simulink model "power_microgrid_v5_battery"  (R2018b)
settings: Solver=ode23tb  StartTime=0.0  StopTime=24*60*60  FixedStep=1/(1000)  MaxStep=60  RelTol=1e-4
PreLoadFcn:
  | load('solar_load_data_24h.mat')
PostLoadFcn:
  | data = xlsread('Domestic_data_all_x3','Sheet1');
  | breakpoints1 = data(2:end,1)'
  | breakpoints2 = data(1,2:end)
  | table_data = data(2:end,2:end)
values from neighbouring files (symbols this model uses):
  SPD_1min = [0 0 0 0 0 0 0 0 0 0 0 0 ... (1441 elements, 1441x1)]    [default_PV_data.mat]
  SPT_1min = [0 60 120 180 240 300 360 420 480 540 600 660 ... (1441 elements, 1441x1)]    [default_PV_data.mat]
libraries: powerlib x155
(part 5 of 5)

== system power_microgrid_v5_battery/PV1 ==
  Clock : Clock
  Complex to Magnitude-Angle : ComplexToMagnitudeAngle  Output=Angle
  Controlled Current Source : powerlib/Electrical Sources/Controlled Current Source  Initialize=on  Source_Type=AC  Amplitude=0  Phase=0  Frequency=50  Measurements=None
      settings: SourceProductName=Simscape Electrical
  Gain10 : Gain  Gain=sqrt(2)
  Gain5 : Gain  Gain=1/230
  Ground2 : powerlib/Elements/Ground  LConnTagsString=a
      settings: SourceProductName=Simscape Electrical
  Magnitude-Angle to Complex1 : MagnitudeAngleToComplex
  Snubber1 : powerlib/Elements/Series RLC Branch  LConnTagsString=__new0  RConnTagsString=__new0  BranchType=R  Resistance=1e6  Inductance=1e-3  SetiL0=off  InitialCurrent=0  Capacitance=1e-6  Setx0=off  InitialVoltage=0  Measurements=None
      settings: SourceProductName=Simscape Electrical
  Solar Data 1-D Lookup Table : Lookup_n-D  NumberOfTableDimensions=1  BreakpointsForDimension1=SPT_1min  BeginIndexSearchUsingPreviousIndexResult=on  Table=SPD_1min  InternalRulePriority=Speed  RndMeth=Simplest  InputSameDT=on
  meas cur3 : powerlib/Measurements/Current Measurement  PhasorSimulation=on  OutputType=Complex  PSBequivalent=0
      settings: SourceProductName=Simscape Electrical
  Conn1 : PMIOPort  Side=Left
  Out1 : Outport
  wires:
  meas cur3/1 -> Out1/1
  Magnitude-Angle to Complex1/1 -> Controlled Current Source/1
  Clock/1 -> Solar Data 1-D Lookup Table/1
  Solar Data 1-D Lookup Table/1 -> Gain5/1
  Gain5/1 -> Gain10/1
  Gain10/1 -> Magnitude-Angle to Complex1/1
  Complex to Magnitude-Angle/1 -> Magnitude-Angle to Complex1/2
  [Vsec] -> Complex to Magnitude-Angle/1
  connections:
  Ground2/LConn1 -- Controlled Current Source/LConn1 -- Snubber1/RConn1
  Snubber1/LConn1 -- Controlled Current Source/RConn1 -- meas cur3/LConn1
  Conn1/RConn1 -- meas cur3/RConn1

== system power_microgrid_v5_battery/PV2 ==
  Clock : Clock
  Complex to Magnitude-Angle : ComplexToMagnitudeAngle  Output=Angle
  Controlled Current Source : powerlib/Electrical Sources/Controlled Current Source  Initialize=on  Source_Type=AC  Amplitude=0  Phase=0  Frequency=50  Measurements=None
      settings: SourceProductName=Simscape Electrical
  Gain10 : Gain  Gain=sqrt(2)
  Gain5 : Gain  Gain=1/230
  Ground2 : powerlib/Elements/Ground  LConnTagsString=a
      settings: SourceProductName=Simscape Electrical
  Magnitude-Angle to Complex1 : MagnitudeAngleToComplex
  Snubber1 : powerlib/Elements/Series RLC Branch  LConnTagsString=__new0  RConnTagsString=__new0  BranchType=R  Resistance=1e6  Inductance=1e-3  SetiL0=off  InitialCurrent=0  Capacitance=1e-6  Setx0=off  InitialVoltage=0  Measurements=None
      settings: SourceProductName=Simscape Electrical
  Solar Data 1-D Lookup Table : Lookup_n-D  NumberOfTableDimensions=1  BreakpointsForDimension1=SPT_1min  BeginIndexSearchUsingPreviousIndexResult=on  Table=SPD_1min  InternalRulePriority=Speed  RndMeth=Simplest  InputSameDT=on
  meas cur3 : powerlib/Measurements/Current Measurement  PhasorSimulation=on  OutputType=Complex  PSBequivalent=0
      settings: SourceProductName=Simscape Electrical
  Conn1 : PMIOPort  Side=Left
  Out1 : Outport
  wires:
  meas cur3/1 -> Out1/1
  Magnitude-Angle to Complex1/1 -> Controlled Current Source/1
  Clock/1 -> Solar Data 1-D Lookup Table/1
  Solar Data 1-D Lookup Table/1 -> Gain5/1
  Gain5/1 -> Gain10/1
  Gain10/1 -> Magnitude-Angle to Complex1/1
  Complex to Magnitude-Angle/1 -> Magnitude-Angle to Complex1/2
  [Vsec] -> Complex to Magnitude-Angle/1
  connections:
  Ground2/LConn1 -- Controlled Current Source/LConn1 -- Snubber1/RConn1
  Snubber1/LConn1 -- Controlled Current Source/RConn1 -- meas cur3/LConn1
  Conn1/RConn1 -- meas cur3/RConn1

== system power_microgrid_v5_battery/PV3 ==
  Clock : Clock
  Complex to Magnitude-Angle : ComplexToMagnitudeAngle  Output=Angle
  Controlled Current Source : powerlib/Electrical Sources/Controlled Current Source  Initialize=on  Source_Type=AC  Amplitude=0  Phase=0  Frequency=50  Measurements=None
      settings: SourceProductName=Simscape Electrical
  Gain10 : Gain  Gain=sqrt(2)
  Gain5 : Gain  Gain=1/230
  Ground2 : powerlib/Elements/Ground  LConnTagsString=a
      settings: SourceProductName=Simscape Electrical
  Magnitude-Angle to Complex1 : MagnitudeAngleToComplex
  Snubber1 : powerlib/Elements/Series RLC Branch  LConnTagsString=__new0  RConnTagsString=__new0  BranchType=R  Resistance=1e6  Inductance=1e-3  SetiL0=off  InitialCurrent=0  Capacitance=1e-6  Setx0=off  InitialVoltage=0  Measurements=None
      settings: SourceProductName=Simscape Electrical
  Solar Data 1-D Lookup Table : Lookup_n-D  NumberOfTableDimensions=1  BreakpointsForDimension1=SPT_1min  BeginIndexSearchUsingPreviousIndexResult=on  Table=SPD_1min  InternalRulePriority=Speed  RndMeth=Simplest  InputSameDT=on
  meas cur3 : powerlib/Measurements/Current Measurement  PhasorSimulation=on  OutputType=Complex  PSBequivalent=0
      settings: SourceProductName=Simscape Electrical
  Conn1 : PMIOPort  Side=Left
  Out1 : Outport
  wires:
  meas cur3/1 -> Out1/1
  Magnitude-Angle to Complex1/1 -> Controlled Current Source/1
  Clock/1 -> Solar Data 1-D Lookup Table/1
  Solar Data 1-D Lookup Table/1 -> Gain5/1
  Gain5/1 -> Gain10/1
  Gain10/1 -> Magnitude-Angle to Complex1/1
  Complex to Magnitude-Angle/1 -> Magnitude-Angle to Complex1/2
  [Vsec] -> Complex to Magnitude-Angle/1
  connections:
  Ground2/LConn1 -- Controlled Current Source/LConn1 -- Snubber1/RConn1
  Snubber1/LConn1 -- Controlled Current Source/RConn1 -- meas cur3/LConn1
  Conn1/RConn1 -- meas cur3/RConn1

== system power_microgrid_v5_battery/PV4 ==
  Clock : Clock
  Complex to Magnitude-Angle : ComplexToMagnitudeAngle  Output=Angle
  Controlled Current Source : powerlib/Electrical Sources/Controlled Current Source  Initialize=on  Source_Type=AC  Amplitude=0  Phase=0  Frequency=50  Measurements=None
      settings: SourceProductName=Simscape Electrical
  Gain10 : Gain  Gain=sqrt(2)
  Gain5 : Gain  Gain=2/230
  Ground2 : powerlib/Elements/Ground  LConnTagsString=a
      settings: SourceProductName=Simscape Electrical
  Magnitude-Angle to Complex1 : MagnitudeAngleToComplex
  Snubber1 : powerlib/Elements/Series RLC Branch  LConnTagsString=__new0  RConnTagsString=__new0  BranchType=R  Resistance=1e6  Inductance=1e-3  SetiL0=off  InitialCurrent=0  Capacitance=1e-6  Setx0=off  InitialVoltage=0  Measurements=None
      settings: SourceProductName=Simscape Electrical
  Solar Data 1-D Lookup Table : Lookup_n-D  NumberOfTableDimensions=1  BreakpointsForDimension1=SPT_1min  BeginIndexSearchUsingPreviousIndexResult=on  Table=SPD_1min  InternalRulePriority=Speed  RndMeth=Simplest  InputSameDT=on
  meas cur3 : powerlib/Measurements/Current Measurement  PhasorSimulation=on  OutputType=Complex  PSBequivalent=0
      settings: SourceProductName=Simscape Electrical
  Conn1 : PMIOPort  Side=Left
  Out1 : Outport
  wires:
  meas cur3/1 -> Out1/1
  Magnitude-Angle to Complex1/1 -> Controlled Current Source/1
  Clock/1 -> Solar Data 1-D Lookup Table/1
  Solar Data 1-D Lookup Table/1 -> Gain5/1
  Gain5/1 -> Gain10/1
  Gain10/1 -> Magnitude-Angle to Complex1/1
  Complex to Magnitude-Angle/1 -> Magnitude-Angle to Complex1/2
  [Vsec] -> Complex to Magnitude-Angle/1
  connections:
  Ground2/LConn1 -- Controlled Current Source/LConn1 -- Snubber1/RConn1
  Snubber1/LConn1 -- Controlled Current Source/RConn1 -- meas cur3/LConn1
  Conn1/RConn1 -- meas cur3/RConn1

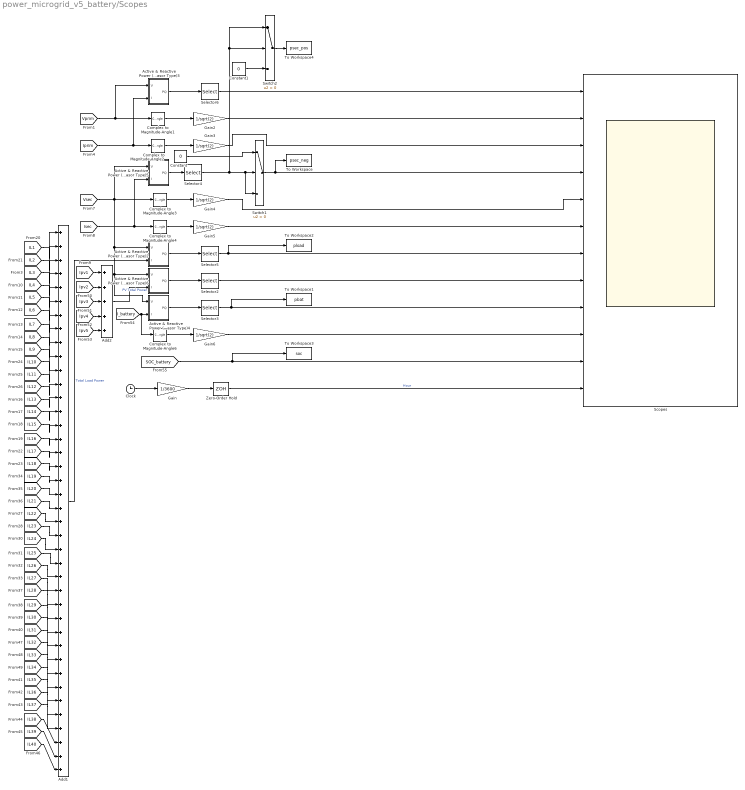
== system power_microgrid_v5_battery/Scopes ==
  Active & Reactive Power (Phasor Type)2 : Subsystem  DialogController=POWERSYS.PowerSysDialog  mask(Active & Reactive Power (Phasor Type)){}
      mask help: Active & Reactive Power (Phasor Type)
      mask init:
      | power_initmask();
      mask Help: This block is part of a subset of blocks in the Extras library that does not have documentation associated with it, other than the block mask description.
      mask Display: disp('')
  Active & Reactive Power (Phasor Type)3 : Subsystem  DialogController=POWERSYS.PowerSysDialog  mask(Active & Reactive Power (Phasor Type)){}
      mask help: Active & Reactive Power (Phasor Type)
      mask init:
      | power_initmask();
      mask Help: This block is part of a subset of blocks in the Extras library that does not have documentation associated with it, other than the block mask description.
      mask Display: disp('')
  Active & Reactive Power (Phasor Type)4 : Subsystem  DialogController=POWERSYS.PowerSysDialog  mask(Active & Reactive Power (Phasor Type)){}
      mask help: Active & Reactive Power (Phasor Type)
      mask init:
      | power_initmask();
      mask Help: This block is part of a subset of blocks in the Extras library that does not have documentation associated with it, other than the block mask description.
      mask Display: disp('')
  Active & Reactive Power (Phasor Type)5 : Subsystem  DialogController=POWERSYS.PowerSysDialog  mask(Active & Reactive Power (Phasor Type)){}
      mask help: Active & Reactive Power (Phasor Type)
      mask init:
      | power_initmask();
      mask Help: This block is part of a subset of blocks in the Extras library that does not have documentation associated with it, other than the block mask description.
      mask Display: disp('')
  Active & Reactive Power (Phasor Type)6 : Subsystem  DialogController=POWERSYS.PowerSysDialog  mask(Active & Reactive Power (Phasor Type)){}
      mask help: Active & Reactive Power (Phasor Type)
      mask init:
      | power_initmask();
      mask Help: This block is part of a subset of blocks in the Extras library that does not have documentation associated with it, other than the block mask description.
      mask Display: disp('')
  Add1 : Sum  Inputs=++++++++++++++++++++++++++++++++++++++++
  Add2 : Sum  Inputs=+++++
  Clock : Clock
  Complex to Magnitude-Angle{1..4,6} (5 alike) : ComplexToMagnitudeAngle  Output=Magnitude
  Constant : Constant  Value=0
  Constant1 : Constant  Value=0
  Gain : Gain  Gain=1/3600
  Gain{2..6} (5 alike) : Gain  Gain=1/sqrt(2)
  Scopes : Scope  NumInputPorts=12
  Selector{2..6} (5 alike) : Selector  InputPortWidth=2  IndexOptions=Index vector (dialog)  Indices=1  OutputSizes=1
  Switch1 : Switch  Criteria=u2 > Threshold
  Switch2 : Switch  Criteria=u2 > Threshold
  To Workspace : ToWorkspace  VariableName=psec_neg  SaveFormat=Timeseries  SampleTime=-1
  To Workspace1 : ToWorkspace  VariableName=pbat  SaveFormat=Timeseries  SampleTime=-1
  To Workspace2 : ToWorkspace  VariableName=pload  SaveFormat=Timeseries  SampleTime=-1
  To Workspace3 : ToWorkspace  VariableName=soc  SaveFormat=Timeseries  SampleTime=-1
  To Workspace4 : ToWorkspace  VariableName=psec_pos  SaveFormat=Timeseries  SampleTime=-1
  Zero-Order Hold : ZeroOrderHold  SampleTime=3600
  wires:
  Clock/1 -> Gain/1
  Gain/1 -> Zero-Order Hold/1
  Gain2/1 -> Scopes/2
  [Vprim] -> Complex to Magnitude-Angle1/1, Active & Reactive Power (Phasor Type)3/1(V)
  [Iprim] -> Complex to Magnitude-Angle2/1, Active & Reactive Power (Phasor Type)3/2(I)
  Gain3/1 -> Scopes/3
  [Vsec] -> Complex to Magnitude-Angle3/1, Active & Reactive Power (Phasor Type)4/1(V), Active & Reactive Power (Phasor Type)6/1(V), Active & Reactive Power (Phasor Type)2/1(V), Active & Reactive Power (Phasor Type)5/1(V)
  Gain4/1 -> Scopes/5
  [Isec] -> Complex to Magnitude-Angle4/1, Active & Reactive Power (Phasor Type)5/2(I)
  Gain5/1 -> Scopes/6
  Selector6/1 -> Scopes/1
  Active & Reactive Power (Phasor Type)3/1(PQ) -> Selector6/1
  Active & Reactive Power (Phasor Type)5/1(PQ) -> Selector4/1
  [IL2] -> Add1/2
  [IL1] -> Add1/1
  [IL3] -> Add1/3
  Active & Reactive Power (Phasor Type)2/1(PQ) -> Selector5/1
  Selector5/1 -> To Workspace2/1, Scopes/7
  Add1/1 -> Active & Reactive Power (Phasor Type)2/2(I)  "Total Load Power"
  Active & Reactive Power (Phasor Type)6/1(PQ) -> Selector2/1
  Selector2/1 -> Scopes/8
  Complex to Magnitude-Angle1/1 -> Gain2/1
  Complex to Magnitude-Angle2/1 -> Gain3/1
  Complex to Magnitude-Angle3/1 -> Gain4/1
  Complex to Magnitude-Angle4/1 -> Gain5/1
  [IL11] -> Add1/11
  [IL10] -> Add1/10
  [IL12] -> Add1/12
  [IL20] -> Add1/20
  [IL19] -> Add1/19
  [IL21] -> Add1/21
  [IL4] -> Add1/4
  [IL5] -> Add1/5
  [IL6] -> Add1/6
  [IL7] -> Add1/7
  [IL8] -> Add1/8
  [IL9] -> Add1/9
  [IL13] -> Add1/13
  [IL14] -> Add1/14
  [IL15] -> Add1/15
  [IL16] -> Add1/16
  [IL17] -> Add1/17
  [IL18] -> Add1/18
  [IL22] -> Add1/22
  [IL23] -> Add1/23
  [IL24] -> Add1/24
  [IL25] -> Add1/25
  [IL26] -> Add1/26
  [IL27] -> Add1/27
  [IL28] -> Add1/28
  [IL29] -> Add1/29
  [IL30] -> Add1/30
  [IL31] -> Add1/31
  [IL32] -> Add1/32
  [IL33] -> Add1/33
  [IL34] -> Add1/34
  [IL35] -> Add1/35
  [IL36] -> Add1/36
  [IL37] -> Add1/37
  [IL38] -> Add1/38
  [IL39] -> Add1/39
  [IL40] -> Add1/40
  [Ipv1] -> Add2/1
  [Ipv2] -> Add2/2
  [Ipv3] -> Add2/3
  Add2/1 -> Active & Reactive Power (Phasor Type)6/2(I)  "PV Total Power"
  [Ipv4] -> Add2/4
  [Ipv5] -> Add2/5
  Zero-Order Hold/1 -> Scopes/12  "Hour"
  Complex to Magnitude-Angle6/1 -> Gain6/1
  [SOC_battery] -> To Workspace3/1, Scopes/11
  Active & Reactive Power (Phasor Type)4/1(PQ) -> Selector3/1
  [I_battery] -> Complex to Magnitude-Angle6/1, Active & Reactive Power (Phasor Type)4/2(I)
  Selector3/1 -> To Workspace1/1, Scopes/9
  Gain6/1 -> Scopes/10
  Selector4/1 -> Switch1/3, Switch1/2, Switch2/1, Switch2/2
  Switch1/1 -> To Workspace/1, Scopes/4
  Constant/1 -> Switch1/1
  Constant1/1 -> Switch2/3
  Switch2/1 -> To Workspace4/1

== system power_microgrid_v5_battery/Subsystem ==
  note: Initial SOC
  note: Integrator
  I_RMS : Inport
  Add : Sum  Inputs=+-
  Constant1 : Constant  Value=0
  Gain : Gain  Gain=1/3600
  Gain3 : Gain  Gain=1/(AH*3600)
  Gain8 : Gain  Gain=100
  Integrator : Integrator
  Battery_Ah : Outport
  Battery_SOC : Outport  Port=2
  wires:
  Integrator/1 -> Gain3/1, Gain/1
  Gain3/1 -> Add/2
  Add/1 -> Gain8/1
  I_RMS/1 -> Integrator/1
  Gain/1 -> Battery_Ah/1
  Gain8/1 -> Battery_SOC/1
  Constant1/1 -> Add/1

== system power_microgrid_v5_battery/Battery_Control/Active & Reactive Power (Phasor Type) ==
  V : Inport
  I : Inport  Port=2
  Complex to Real-Imag : ComplexToRealImag
  K : Gain  Gain=1/2  SaturateOnIntegerOverflow=on  OutDataTypeStr=Inherit: Same as input  ParamDataTypeStr=Inherit: Same as input
  Math Function : Math  Operator=conj  SaturateOnIntegerOverflow=on
  Mux : Mux  Inputs=2
  Product2 : Product  SaturateOnIntegerOverflow=on  InputSameDT=on  OutDataTypeStr=Inherit: Same as first input
  PQ : Outport
  wires:
  Mux/1 -> PQ/1
  Complex to Real-Imag/2 -> Mux/2
  Complex to Real-Imag/1 -> Mux/1
  V/1 -> Product2/1
  Math Function/1 -> Product2/2
  Product2/1 -> K/1
  K/1 -> Complex to Real-Imag/1
  I/1 -> Math Function/1

== system power_microgrid_v5_battery/Battery_Control/Subsystem ==
  In1 : Inport
  Integral Gain : Gain  Gain=-0.1
  Integrator : Integrator  LimitOutput=on  UpperSaturationLimit=50  LowerSaturationLimit=-50
  Out1 : Outport
  wires:
  Integrator/1 -> Out1/1
  In1/1 -> Integral Gain/1
  Integral Gain/1 -> Integrator/1

== system power_microgrid_v5_battery/Scopes/Active & Reactive Power (Phasor Type)2 ==
  V : Inport
  I : Inport  Port=2
  Complex to Real-Imag : ComplexToRealImag
  K : Gain  Gain=1/2  SaturateOnIntegerOverflow=on  OutDataTypeStr=Inherit: Same as input  ParamDataTypeStr=Inherit: Same as input
  Math Function : Math  Operator=conj  SaturateOnIntegerOverflow=on
  Mux : Mux  Inputs=2
  Product2 : Product  SaturateOnIntegerOverflow=on  InputSameDT=on  OutDataTypeStr=Inherit: Same as first input
  PQ : Outport
  wires:
  Mux/1 -> PQ/1
  Complex to Real-Imag/2 -> Mux/2
  Complex to Real-Imag/1 -> Mux/1
  V/1 -> Product2/1
  Math Function/1 -> Product2/2
  Product2/1 -> K/1
  K/1 -> Complex to Real-Imag/1
  I/1 -> Math Function/1

== system power_microgrid_v5_battery/Scopes/Active & Reactive Power (Phasor Type)3 ==
  V : Inport
  I : Inport  Port=2
  Complex to Real-Imag : ComplexToRealImag
  K : Gain  Gain=1/2  SaturateOnIntegerOverflow=on  OutDataTypeStr=Inherit: Same as input  ParamDataTypeStr=Inherit: Same as input
  Math Function : Math  Operator=conj  SaturateOnIntegerOverflow=on
  Mux : Mux  Inputs=2
  Product2 : Product  SaturateOnIntegerOverflow=on  InputSameDT=on  OutDataTypeStr=Inherit: Same as first input
  PQ : Outport
  wires:
  Mux/1 -> PQ/1
  Complex to Real-Imag/2 -> Mux/2
  Complex to Real-Imag/1 -> Mux/1
  V/1 -> Product2/1
  Math Function/1 -> Product2/2
  Product2/1 -> K/1
  K/1 -> Complex to Real-Imag/1
  I/1 -> Math Function/1

== system power_microgrid_v5_battery/Scopes/Active & Reactive Power (Phasor Type)4 ==
  V : Inport
  I : Inport  Port=2
  Complex to Real-Imag : ComplexToRealImag
  K : Gain  Gain=1/2  SaturateOnIntegerOverflow=on  OutDataTypeStr=Inherit: Same as input  ParamDataTypeStr=Inherit: Same as input
  Math Function : Math  Operator=conj  SaturateOnIntegerOverflow=on
  Mux : Mux  Inputs=2
  Product2 : Product  SaturateOnIntegerOverflow=on  InputSameDT=on  OutDataTypeStr=Inherit: Same as first input
  PQ : Outport
  wires:
  Mux/1 -> PQ/1
  Complex to Real-Imag/2 -> Mux/2
  Complex to Real-Imag/1 -> Mux/1
  V/1 -> Product2/1
  Math Function/1 -> Product2/2
  Product2/1 -> K/1
  K/1 -> Complex to Real-Imag/1
  I/1 -> Math Function/1

== system power_microgrid_v5_battery/Scopes/Active & Reactive Power (Phasor Type)5 ==
  V : Inport
  I : Inport  Port=2
  Complex to Real-Imag : ComplexToRealImag
  K : Gain  Gain=1/2  SaturateOnIntegerOverflow=on  OutDataTypeStr=Inherit: Same as input  ParamDataTypeStr=Inherit: Same as input
  Math Function : Math  Operator=conj  SaturateOnIntegerOverflow=on
  Mux : Mux  Inputs=2
  Product2 : Product  SaturateOnIntegerOverflow=on  InputSameDT=on  OutDataTypeStr=Inherit: Same as first input
  PQ : Outport
  wires:
  Mux/1 -> PQ/1
  Complex to Real-Imag/2 -> Mux/2
  Complex to Real-Imag/1 -> Mux/1
  V/1 -> Product2/1
  Math Function/1 -> Product2/2
  Product2/1 -> K/1
  K/1 -> Complex to Real-Imag/1
  I/1 -> Math Function/1

== system power_microgrid_v5_battery/Scopes/Active & Reactive Power (Phasor Type)6 ==
  V : Inport
  I : Inport  Port=2
  Complex to Real-Imag : ComplexToRealImag
  K : Gain  Gain=1/2  SaturateOnIntegerOverflow=on  OutDataTypeStr=Inherit: Same as input  ParamDataTypeStr=Inherit: Same as input
  Math Function : Math  Operator=conj  SaturateOnIntegerOverflow=on
  Mux : Mux  Inputs=2
  Product2 : Product  SaturateOnIntegerOverflow=on  InputSameDT=on  OutDataTypeStr=Inherit: Same as first input
  PQ : Outport
  wires:
  Mux/1 -> PQ/1
  Complex to Real-Imag/2 -> Mux/2
  Complex to Real-Imag/1 -> Mux/1
  V/1 -> Product2/1
  Math Function/1 -> Product2/2
  Product2/1 -> K/1
  K/1 -> Complex to Real-Imag/1
  I/1 -> Math Function/1
